simulink model "System_Design_Quadrocopter_2012"  (Simulink 8.1)
settings: Solver=ode45  StartTime=0.0  StopTime=inf  RelTol=1e-3
PostLoadFcn:
  | Reglerauslegung
values from neighbouring files (symbols this model uses):
  f1 = (I_y-I_z)/I_x    [quadrocopter_param.m]
  f2 = rot.J_z/I_x    [quadrocopter_param.m]
  f3 = (I_z-I_x)/I_y    [quadrocopter_param.m]
  f4 = rot.J_z/I_y    [quadrocopter_param.m]
  f5 = (I_x-I_y)/I_z    [quadrocopter_param.m]
  g = 9.81    [quadrocopter_param.m]
  I_x = elec.I_x+bat.I_x+2*boom.I_1x+2*boom.I_1y+2*mot.I_1x+2*mot.I_1y+                             2*rot.I_1x+2*rot.I_1y    [quadrocopter_param.m]
  I_y = elec.I_y+bat.I_y+2*boom.I_1x+2*boom.I_1y+2*mot.I_1x+2*mot.I_1y+                             2*rot.I_1x+2*rot.I_1y    [quadrocopter_param.m]
  I_z = elec.I_z+bat.I_z+4*boom.I_1z+4*mot.I_1z+4*rot.I_1z    [quadrocopter_param.m]
  m = m*1.2    [quadrocopter_param.m]
  r_psi0 = 0    [quadrocopter_param.m]
  r_theta0 = 0    [quadrocopter_param.m]
  theta0 = 0    [quadrocopter_param.m]
  Ts = 0.005    [quadrocopter_param.m]
undefined symbols (not defined in the file or in its folder): boom, K_ret, KV
libraries: Copter_Library x6, simulink x6, dspobslib x4
settings Model: Creator=roczit00  LastModifiedBy=Agrawal
settings DebuggingCC: AlgebraicLoopMsg=none  SolverPrmCheckMsg=none  UnconnectedInputMsg=none  UnconnectedOutputMsg=none  UnconnectedLineMsg=none
settings SFSimCC: SimParseCustomCode=off

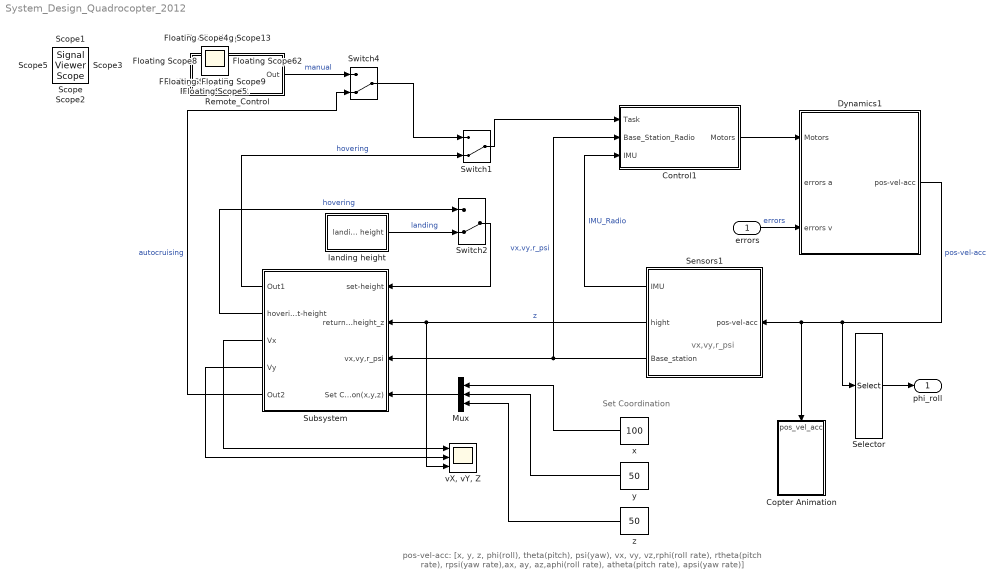
== system System_Design_Quadrocopter_2012 ==
  note: pos-vel-acc: [x, y, z, phi(roll), theta(pitch), psi(yaw), vx, vy, vz,rphi(roll rate), rtheta(pitch rate), rpsi(yaw rate),ax, ay, az,aphi(roll rate), atheta(pitch rate), apsi(yaw rate)]
  note: vx,vy,r_psi
  note: Set Coordination
  errors : Inport
  Control1 : Subsystem
  Copter Animation : Subsystem  mask(Quadrocopter Animation){AXES=[-200 200 -200 200 0 200], T_INT=1/25, K_VAR=Feste Position, K_POS=[200 200 0], K_ANGLE=27, A_ON=on, u_phi=on, u_theta=on, u_psi=on, u_x=on, u_y=on, u_z=on}
      mask prompts: AXES "Achsen Grenzen [xmin xmax ymin ymax zmin zmax]"; T_INT "Zeitintervall zwischen Aktualisierungen [s]:"; K_VAR "Kamera Art:"; K_POS "Ort der Kamera [xc yc zc]:"; K_ANGLE "Öffnungswinkel der Kamera [Grad]:"; A_ON "Animation Einschalten:"; u_phi "Use Input phi:"; u_theta "Use Input theta:"; u_psi "Use Input psi:"; u_x "Use Input x:"; u_y "Use Input y:"; u_z "Use Input z:"
      mask help: Erstellt eine 3-D animierte Ansicht eines Quadrocopters.
      mask init:
      | Config.axes = AXES;
      | Config.update = T_INT;
      | Config.camera_view = K_VAR;
      | Config.camera_pos = K_POS;
      | Config.view = K_ANGLE;
      | Config.Animenable = A_ON;
      | Config.phi = u_phi;
      | Config.theta = u_theta;
      | Config.psi = u_psi;
      | Config.x = u_x;
      | Config.y = u_y;
      | Config.z = u_z;
      mask Help:
      | <p>Dieser Block erstellt ein 3 dimensionales Fenster eines Quadrocopters.
      | 
      | <p><H4>Block Eingänge</H4>
      | Der Eingangsvektor bestehend aus:
      | <ul>
      | <li>X-Koordinate - Ort bezogen auf die X-Achse
      | <li>Y-Koordinate - Ort bezogen auf die Y-Achse
      | <li>Z-Koordinate - Ort bezogen auf die Z-Achse
      | <li>Psi - Yaw Drehung um die Z-Achse
      | <li>Phi - Roll Drehen um die Achse in Flugrichtung
      | <li>theta - pitch Neigung in Flugrichtung nach oben bzw. unten
      | </ul></p>
      mask TypeOptions K_VAR: Feste Position | Frei bewegbar
  Dynamics1 : Subsystem
  Mux : Mux  Inputs=3
  Remote_Control : Subsystem
  Selector : Selector  InputPortWidth=19  IndexOptions=Index vector (dialog)  Indices=[4 5]  OutputSizes=1
  Sensors1 : Subsystem
  Subsystem : Subsystem
  Switch1 : ManualSwitch  CurrentSetting=0
  Switch2 : ManualSwitch  CurrentSetting=0
  Switch4 : ManualSwitch  CurrentSetting=0
  landing height : Subsystem
  "vX, vY, Z" : Scope  NumInputPorts=3
      settings: TimeRange=70  YMin=-5~-10~-20  YMax=25~20~100  SaveName=ScopeData31
  x : Constant  Value=100
  y : Constant  Value=50
  z : Constant  Value=50
  phi_roll : Outport
  Floating Scope{,1..13} (14 alike) : Scope
      Floating Scope settings: Floating=on  YMin=-40  YMax=90
      Floating Scope1 settings: Floating=on
      Floating Scope10 settings: Floating=on  SaveName=ScopeData12
      Floating Scope11 settings: Floating=on  SaveName=ScopeData13
      Floating Scope12 settings: Floating=on  YMin=-2500  YMax=27500  SaveName=ScopeData14
      Floating Scope13 settings: Floating=on  YMin=0  YMax=0.3  SaveName=ScopeData15
      Floating Scope2 settings: Floating=on  YMin=-6000  YMax=2500  SaveName=ScopeData2
      Floating Scope3 settings: Floating=on  SaveName=ScopeData3
      Floating Scope4 settings: Floating=on  SaveName=ScopeData4
      Floating Scope5 settings: Floating=on  YMin=-0.7  YMax=0.8  SaveName=ScopeData5
      Floating Scope6 settings: Floating=on  YMin=-1  YMax=1  SaveName=ScopeData6
      Floating Scope7 settings: Floating=on  YMin=-15  YMax=10  SaveName=ScopeData7
      Floating Scope8 settings: Floating=on  YMax=45  SaveName=ScopeData10
      Floating Scope9 settings: Floating=on  YMin=-7  YMax=9  SaveName=ScopeData11
  Scope{,1..3,5} (5 alike) : SignalViewerScope  IOType=viewer  RefreshTime=0.035000
      Scope settings: YMin=-0.01  YMax=0.1
      Scope2 settings: SaveName=ScopeData2
      Scope3 settings: SaveName=ScopeData3
      Scope5 settings: YMin=0  YMax=275  SaveName=ScopeData4
  wires:
  Dynamics1/1(pos-vel-acc) -> Selector/1, Sensors1/1(pos-vel-acc), Copter Animation/1(pos_vel_acc)  "pos-vel-acc"
  Sensors1/1(IMU) -> Control1/3(IMU)  "IMU_Radio"
  Sensors1/3(Base_station) -> Control1/2(Base_Station_Radio), Subsystem/3(vx,vy,r_psi)  "vx,vy,r_psi"
  errors/1 -> Dynamics1/3(errors v)  "errors"
  Selector/1 -> phi_roll/1
  Control1/1(Motors) -> Dynamics1/1(Motors)
  Subsystem/1(Out1) -> Switch1/2  "hovering"
  Switch1/1 -> Control1/1(Task)
  Sensors1/2(hight) -> Subsystem/2(return height_z), "vX, vY, Z"/3  "z"
  Switch2/1 -> Subsystem/1(set-height)
  Subsystem/3(Vx) -> "vX, vY, Z"/1
  Subsystem/4(Vy) -> "vX, vY, Z"/2
  landing height/1(landing height) -> Switch2/2  "landing"
  Subsystem/2(hovering set-height) -> Switch2/1  "hovering"
  Switch4/1 -> Switch1/1
  Remote_Control/1(Out) -> Switch4/1  "manual"
  Subsystem/5(Out2) -> Switch4/2  "autocruising"
  x/1 -> Mux/1
  y/1 -> Mux/2
  z/1 -> Mux/3
  Mux/1 -> Subsystem/4(Set Coordination(x,y,z))

== system System_Design_Quadrocopter_2012/Control1 ==
  Task : Inport  OutDataTypeStr=double  PortDimensions=4
  Base_Station_Radio : Inport  Port=2
  IMU : Inport  Port=3
  Mux : Mux  Inputs=2
  Mux1 : Mux  Inputs=2
  State Space - 2nd approach : Subsystem
  Motors : Outport  PortDimensions=4
  wires:
  IMU/1 -> Mux/1  "[ax, ay, r_phi, r_theta,r_psi]"
  Task/1 -> Mux/2  "[phi(roll), theta(pitch),rpsi(yaw rate), T(thrust)]"
  Mux/1 -> Mux1/1
  Base_Station_Radio/1 -> Mux1/2  "[vx, vy, rpsi, vz]"
  Mux1/1 -> State Space - 2nd approach/1(In1)
  State Space - 2nd approach/1(Out1) -> Motors/1

== system System_Design_Quadrocopter_2012/Copter Animation ==
  pos_vel_acc : Inport  PortDimensions=19
  S-Function : S-Function  FunctionName=Copter_Animation  Parameters=Config  EnableBusSupport=off
  Selector2 : Selector  InputPortWidth=19  IndexOptions=Index vector (dialog)  Indices=[1 2 3 4 5 6]  OutputSizes=1
  wires:
  pos_vel_acc/1 -> Selector2/1
  Selector2/1 -> S-Function/1

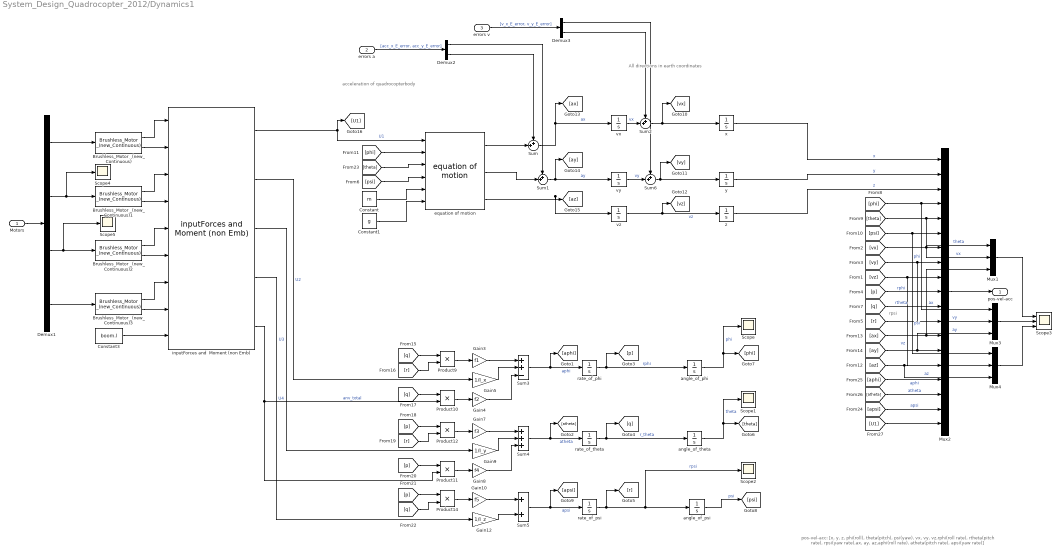
== system System_Design_Quadrocopter_2012/Dynamics1 ==
  note: rpsi
  note: pos-vel-acc: [x, y, z, phi(roll), theta(pitch), psi(yaw), vx, vy, vz,rphi(roll rate), rtheta(pitch rate), rpsi(yaw rate),ax, ay, az,aphi(roll rate), atheta(pitch rate), apsi(yaw rate)]
  note: All directions in earth coordinates
  note: acceleration of quadrocopterbody
  Motors : Inport
  errors a : Inport  Port=2
  errors v : Inport  Port=3
  Brushless_Motor _(new_Continuous){,1..3} (4 alike) : Copter_Library/Brushless_Motor _(new_Continuous)  M_error=0.99
  Constant : Constant  Value=m
  Constant1 : Constant  Value=g
  Constant3 : Constant  Value=boom.l
  Demux1 : Demux
  Demux2 : Demux  Outputs=2
  Demux3 : Demux  Outputs=2
  Gain10 : Gain  Gain=f5
  Gain12 : Gain  Gain=1/I_z
  Gain3 : Gain  Gain=f1
  Gain4 : Gain  Gain=f2
  Gain5 : Gain  Gain=1/I_x
  Gain7 : Gain  Gain=f3
  Gain8 : Gain  Gain=f4
  Gain9 : Gain  Gain=1/I_y
  Mux1 : Mux  Inputs=3
  Mux2 : Mux  Inputs=19
  Mux3 : Mux  Inputs=3
  Mux4 : Mux  Inputs=3
  Product{9..12,14} (5 alike) : Product  RndMeth=Zero
  Scope{,1..2,4..5} (5 alike) : Scope
      Scope settings: YMin=-1  YMax=1  SaveName=ScopeData8
      Scope1 settings: YMin=-54  YMax=-49.5  SaveName=ScopeData9
      Scope2 settings: YMin=17.1  YMax=19.1  SaveName=ScopeData16
      Scope4 settings: YMin=-1  YMax=260  SaveName=ScopeData18
      Scope5 settings: YMin=-1  YMax=260  SaveName=ScopeData19
  Scope3 : Scope  NumInputPorts=3
      settings: TimeRange=10  YMin=-5~-5~-10  YMax=8~7~40  SaveName=ScopeData29
  Sum{,1..2,6} (4 alike) : Sum  Inputs=++|
  Sum3 : Sum  Inputs=++-
  Sum4 : Sum  Inputs=+++
  Sum5 : Sum
  angle_of_phi : Integrator
  angle_of_psi : Integrator
  angle_of_theta : Integrator  InitialCondition=theta0
  equation of motion : Copter_Library/equation of motion
  inputForces and  Moment (non Emb) : Copter_Library/inputForces and  Moment (non Emb)
  rate_of_phi : Integrator
  rate_of_psi : Integrator  InitialCondition=r_psi0
  rate_of_theta : Integrator  InitialCondition=r_theta0
  vx : Integrator
  vy : Integrator
  vz : Integrator
  x : Integrator
  y : Integrator
  z : Integrator
  pos-vel-acc : Outport
  wires:
  [apsi] -> Mux2/18  "apsi"
  [atheta] -> Mux2/17  "atheta"
  [aphi] -> Mux2/16  "aphi"
  [az] -> Mux2/15, Mux4/3  "az"
  [ay] -> Mux2/14, Mux3/3  "ay"
  [ax] -> Mux2/13, Mux1/3  "ax"
  [r] -> Mux2/12
  [q] -> Mux2/11  "rtheta"
  [p] -> Mux2/10  "rphi"
  [vz] -> Mux2/9, Mux4/2  "vz"
  [vy] -> Mux2/8, Mux3/2  "vy"
  [vx] -> Mux2/7, Mux1/2  "vx"
  [psi] -> Mux2/6, Mux4/1  "psi"
  [theta] -> Mux2/5, Mux1/1  "theta"
  [phi] -> Mux2/4, Mux3/1  "phi"
  z/1 -> Mux2/3  "z"
  Mux2/1 -> pos-vel-acc/1
  errors a/1 -> Demux2/1  "[acc_x_E_error, acc_y_E_error]"
  Motors/1 -> Demux1/1
  Demux1/3 -> Brushless_Motor _(new_Continuous)2/1, Scope5/1
  Demux1/4 -> Brushless_Motor _(new_Continuous)3/1
  Demux1/2 -> Brushless_Motor _(new_Continuous)1/1, Scope4/1
  Demux1/1 -> Brushless_Motor _(new_Continuous)/1
  vz/1 -> [vz], z/1  "vz"
  Constant3/1 -> inputForces and  Moment (non Emb)/9
  Sum5/1 -> [apsi], rate_of_psi/1  "apsi"
  inputForces and  Moment (non Emb)/4 -> Gain12/1  "U4"
  Gain12/1 -> Sum5/2
  Gain10/1 -> Sum5/1
  Product14/1 -> Gain10/1
  [q] -> Product14/2
  [p] -> Product14/1
  Sum4/1 -> [atheta], rate_of_theta/1  "atheta"
  inputForces and  Moment (non Emb)/3 -> Gain9/1  "U3"
  Gain8/1 -> Sum4/3
  Gain9/1 -> Sum4/2
  Product11/1 -> Gain8/1
  [p] -> Product11/1
  Gain7/1 -> Sum4/1
  Product12/1 -> Gain7/1
  [r] -> Product12/2
  [p] -> Product12/1
  Sum3/1 -> [aphi], rate_of_phi/1  "aphi"
  Gain4/1 -> Sum3/3
  Gain5/1 -> Sum3/2
  inputForces and  Moment (non Emb)/2 -> Gain5/1  "U2"
  Product10/1 -> Gain4/1
  [q] -> Product10/1
  Gain3/1 -> Sum3/1
  Product9/1 -> Gain3/1
  [r] -> Product9/2
  [q] -> Product9/1
  inputForces and  Moment (non Emb)/5 -> Product11/2, Product10/2  "anv_total"
  angle_of_phi/1 -> [phi], Scope/1  "phi"
  angle_of_theta/1 -> [theta], Scope1/1  "theta"
  angle_of_psi/1 -> [psi]  "psi"
  rate_of_phi/1 -> [p], angle_of_phi/1  "rphi"
  rate_of_theta/1 -> angle_of_theta/1, [q]  "r_theta"
  rate_of_psi/1 -> [r], angle_of_psi/1, Scope2/1  "rpsi"
  Brushless_Motor _(new_Continuous)/1 -> inputForces and  Moment (non Emb)/1
  Brushless_Motor _(new_Continuous)/2 -> inputForces and  Moment (non Emb)/2
  Brushless_Motor _(new_Continuous)1/1 -> inputForces and  Moment (non Emb)/3
  Brushless_Motor _(new_Continuous)1/2 -> inputForces and  Moment (non Emb)/4
  Brushless_Motor _(new_Continuous)2/1 -> inputForces and  Moment (non Emb)/5
  Brushless_Motor _(new_Continuous)2/2 -> inputForces and  Moment (non Emb)/6
  Brushless_Motor _(new_Continuous)3/1 -> inputForces and  Moment (non Emb)/7
  Brushless_Motor _(new_Continuous)3/2 -> inputForces and  Moment (non Emb)/8
  x/1 -> Mux2/1  "x"
  y/1 -> Mux2/2  "y"
  Sum1/1 -> [ay], vy/1  "ay"
  Sum/1 -> [ax], vx/1  "ax"
  Demux2/2 -> Sum/1
  Demux2/1 -> Sum1/1
  equation of motion/3 -> [az], vz/1
  equation of motion/2 -> Sum1/2
  equation of motion/1 -> Sum/2
  inputForces and  Moment (non Emb)/1 -> [U1], equation of motion/1  "U1"
  [phi] -> equation of motion/2
  [theta] -> equation of motion/3
  [psi] -> equation of motion/4
  Constant/1 -> equation of motion/5
  Constant1/1 -> equation of motion/6
  [U1] -> Mux2/19
  errors v/1 -> Demux3/1  "[v_x_E_error, v_y_E_error]"
  Demux3/2 -> Sum2/1
  Demux3/1 -> Sum6/1
  vx/1 -> Sum2/2  "vx"
  Sum2/1 -> [vx], x/1
  vy/1 -> Sum6/2  "vy"
  Sum6/1 -> [vy], y/1
  Mux1/1 -> Scope3/1
  Mux3/1 -> Scope3/2
  Mux4/1 -> Scope3/3

== system System_Design_Quadrocopter_2012/Remote_Control ==
  3D-Mouse : ManualSwitch  CurrentSetting=0
  Allow 3D Mouse : dspobslib/DSP Constant  Value=1  SampleMode=Discrete  discreteOutput=Sample-based  continuousOutput=Sample-based  sampTime=inf  framePeriod=2  dataType=boolean  isSigned=on  wordLen=16  udDataType=sfix(16)  fracBitsMode=Best precision  numFracBits=15  InterpretAs1D=-inf  Ts=-inf  FramebasedOutput=-inf
  Disable 3D Mouse : dspobslib/DSP Constant  Value=0  SampleMode=Discrete  discreteOutput=Sample-based  continuousOutput=Sample-based  sampTime=inf  framePeriod=2  dataType=boolean  isSigned=on  wordLen=16  udDataType=sfix(16)  fracBitsMode=Best precision  numFracBits=15  InterpretAs1D=-inf  Ts=-inf  FramebasedOutput=-inf
  Manual Switch2 : ManualSwitch
  Remote_Control_3d_mouse : Subsystem  AncestorBlock=Remote_Control_Library/Remote_Control_3d_mouse
  Remote_Control_setting : Subsystem  AncestorBlock=Remote_Control_Library/Remote_Control_Pitch_stimuli
  Out : Outport
  wires:
  Remote_Control_setting/1(Out) -> Manual Switch2/1
  Manual Switch2/1 -> Out/1
  Allow 3D Mouse/1 -> 3D-Mouse/1
  Disable 3D Mouse/1 -> 3D-Mouse/2
  3D-Mouse/1 -> Remote_Control_3d_mouse/Enable
  Remote_Control_3d_mouse/1(Out1) -> Manual Switch2/2

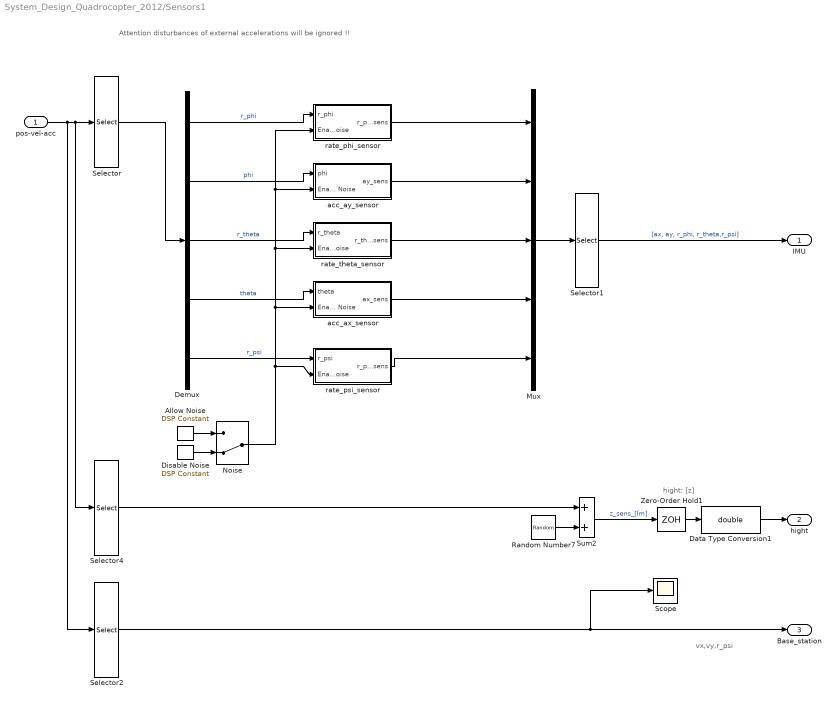
== system System_Design_Quadrocopter_2012/Sensors1 ==
  note: Attention disturbances of external accelerations will be ignored !!
  note: hight: [z]
  note: vx,vy,r_psi
  pos-vel-acc : Inport  PortDimensions=19
  Allow Noise : dspobslib/DSP Constant  Value=1  SampleMode=Discrete  discreteOutput=Sample-based  continuousOutput=Sample-based  sampTime=inf  framePeriod=2  dataType=boolean  isSigned=on  wordLen=16  udDataType=sfix(16)  fracBitsMode=Best precision  numFracBits=15  InterpretAs1D=-inf  Ts=-inf  FramebasedOutput=-inf
  Data Type Conversion1 : DataTypeConversion  OutDataTypeStr=double  RndMeth=Round
  Demux : Demux  Outputs=5
  Disable Noise : dspobslib/DSP Constant  Value=0  SampleMode=Discrete  discreteOutput=Sample-based  continuousOutput=Sample-based  sampTime=inf  framePeriod=2  dataType=boolean  isSigned=on  wordLen=16  udDataType=sfix(16)  fracBitsMode=Best precision  numFracBits=15  InterpretAs1D=-inf  Ts=-inf  FramebasedOutput=-inf
  Mux : Mux  Inputs=5
  Noise : ManualSwitch  CurrentSetting=0
  Random Number7 : RandomNumber  Variance=3.0462e-8  Seed=5756  SampleTime=0.01
  Scope : Scope
      settings: SaveName=ScopeData30
  Selector : Selector  InputPortWidth=19  IndexOptions=Index vector (dialog)  Indices=[10 4 11 5 12]  OutputSizes=1
  Selector1 : Selector  InputPortWidth=5  IndexOptions=Index vector (dialog)  Indices=[4 2 1 3 5]  OutputSizes=1
  Selector2 : Selector  InputPortWidth=19  IndexOptions=Index vector (dialog)  Indices=[7 8 12]  OutputSizes=1
  Selector4 : Selector  InputPortWidth=19  IndexOptions=Index vector (dialog)  Indices=[3]  OutputSizes=1
  Sum2 : Sum
  Zero-Order Hold1 : ZeroOrderHold  SampleTime=Ts
  acc_ax_sensor : Subsystem
  acc_ay_sensor : Subsystem
  rate_phi_sensor : Subsystem
  rate_psi_sensor : Subsystem
  rate_theta_sensor : Subsystem
  IMU : Outport
  hight : Outport  Port=2
  Base_station : Outport  Port=3
  wires:
  pos-vel-acc/1 -> Selector/1, Selector4/1, Selector2/1
  Selector/1 -> Demux/1
  rate_phi_sensor/1(r_phi_sens) -> Mux/1
  acc_ay_sensor/1(ay_sens) -> Mux/2
  rate_theta_sensor/1(r_theta_sens) -> Mux/3
  acc_ax_sensor/1(ax_sens) -> Mux/4
  rate_psi_sensor/1(r_psi_sens) -> Mux/5
  Demux/1 -> rate_phi_sensor/1(r_phi)  "r_phi"
  Demux/2 -> acc_ay_sensor/1(phi)  "phi"
  Demux/3 -> rate_theta_sensor/1(r_theta)  "r_theta"
  Demux/4 -> acc_ax_sensor/1(theta)  "theta"
  Demux/5 -> rate_psi_sensor/1(r_psi)  "r_psi"
  Mux/1 -> Selector1/1
  Selector1/1 -> IMU/1  "[ax, ay, r_phi, r_theta,r_psi]"
  Allow Noise/1 -> Noise/1
  Disable Noise/1 -> Noise/2
  Noise/1 -> rate_psi_sensor/2(Enable Noise), acc_ax_sensor/2(Enable Noise), rate_theta_sensor/2(Enable Noise), acc_ay_sensor/2(Enable Noise), rate_phi_sensor/2(Enable Noise)
  Random Number7/1 -> Sum2/2
  Selector4/1 -> Sum2/1
  Sum2/1 -> Zero-Order Hold1/1  "z_sens_[Ïm]"
  Zero-Order Hold1/1 -> Data Type Conversion1/1
  Data Type Conversion1/1 -> hight/1
  Selector2/1 -> Base_station/1, Scope/1

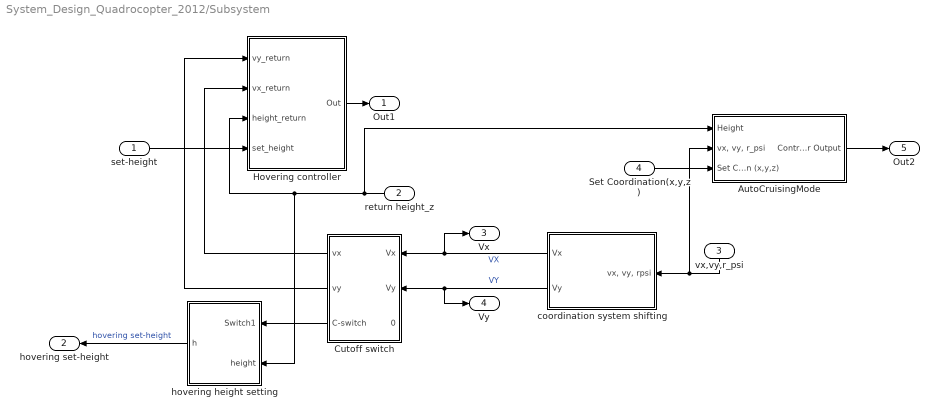
== system System_Design_Quadrocopter_2012/Subsystem ==
  set-height : Inport
  return height_z : Inport  Port=2
  vx,vy,r_psi : Inport  Port=3
  Set Coordination(x,y,z) : Inport  Port=4
  AutoCruisingMode : Subsystem
  Cutoff switch : Subsystem
  Hovering controller : Subsystem
  coordination system shifting : Subsystem
  hovering height setting : MATLAB Function  TreatAsAtomicUnit=on
  Out1 : Outport
  hovering set-height : Outport  Port=2
  Vx : Outport  Port=3
  Vy : Outport  Port=4
  Out2 : Outport  Port=5
  wires:
  Cutoff switch/3(C-switch) -> hovering height setting/1(Switch1)
  coordination system shifting/2(Vy) -> Cutoff switch/2(Vy), Vy/1  "VY"
  Cutoff switch/1(vx) -> Hovering controller/2(vx_return)
  Cutoff switch/2(vy) -> Hovering controller/1(vy_return)
  return height_z/1 -> Hovering controller/3(height_return), hovering height setting/2(height), AutoCruisingMode/1(Height)
  vx,vy,r_psi/1 -> coordination system shifting/1("vx, vy, rpsi"), AutoCruisingMode/2("vx, vy, r_psi")
  Hovering controller/1(Out) -> Out1/1
  set-height/1 -> Hovering controller/4(set_height)
  hovering height setting/1(h) -> hovering set-height/1  "hovering set-height"
  coordination system shifting/1(Vx) -> Cutoff switch/1(Vx), Vx/1  "VX"
  AutoCruisingMode/1(Controller Output) -> Out2/1
  Set Coordination(x,y,z)/1 -> AutoCruisingMode/3(Set Coordination (x,y,z))

== system System_Design_Quadrocopter_2012/landing height ==
  Add1 : Sum
  Compensate height : Constant  Value=5
  landing set_height : Constant  Value=10
  landing height : Outport
  wires:
  landing set_height/1 -> Add1/2
  Compensate height/1 -> Add1/1
  Add1/1 -> landing height/1

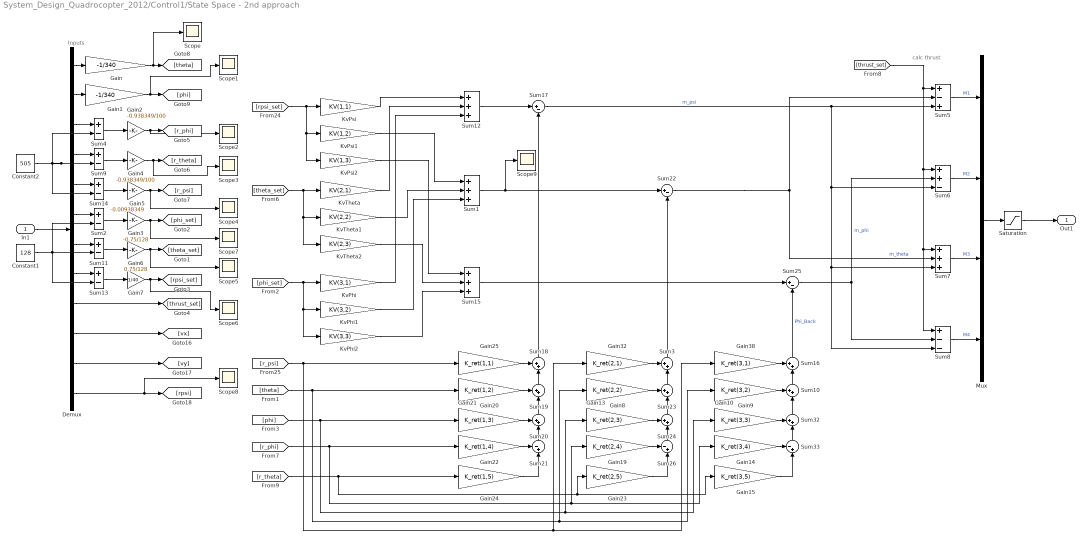
== system System_Design_Quadrocopter_2012/Control1/State Space - 2nd approach ==
  note: calc thrust
  note: Inputs
  In1 : Inport
  Constant1 : Constant  Value=128
  Constant2 : Constant  Value=505
  Demux : Demux  Outputs=12
  Gain : Gain  Gain=-1/340
  Gain1 : Gain  Gain=-1/340
  Gain10 : Gain  Gain=K_ret(3,3)
  Gain13 : Gain  Gain=K_ret(2,3)
  Gain14 : Gain  Gain=K_ret(3,4)
  Gain15 : Gain  Gain=K_ret(3,5)
  Gain19 : Gain  Gain=K_ret(2,4)
  Gain2 : Gain  Gain=-0.938349/100
  Gain20 : Gain  Gain=K_ret(1,2)
  Gain21 : Gain  Gain=K_ret(1,3)
  Gain22 : Gain  Gain=K_ret(1,4)
  Gain23 : Gain  Gain=K_ret(2,5)
  Gain24 : Gain  Gain=K_ret(1,5)
  Gain25 : Gain  Gain=K_ret(1,1)
  Gain3 : Gain  Gain=-0.75/128
  Gain32 : Gain  Gain=K_ret(2,1)
  Gain38 : Gain  Gain=K_ret(3,1)
  Gain4 : Gain  Gain=-0.938349/100
  Gain5 : Gain  Gain=-0.00938349
  Gain6 : Gain  Gain=0.75/128
  Gain7 : Gain  Gain=1/40
  Gain8 : Gain  Gain=K_ret(2,2)
  Gain9 : Gain  Gain=K_ret(3,2)
  KvPhi : Gain  Gain=KV(3,1)
  KvPhi1 : Gain  Gain=KV(3,2)
  KvPhi2 : Gain  Gain=KV(3,3)
  KvPsi : Gain  Gain=KV(1,1)
  KvPsi1 : Gain  Gain=KV(1,2)
  KvPsi2 : Gain  Gain=KV(1,3)
  KvTheta : Gain  Gain=KV(2,1)
  KvTheta1 : Gain  Gain=KV(2,2)
  KvTheta2 : Gain  Gain=KV(2,3)
  Mux : Mux
  Saturation : Saturate  UpperLimit=255  LowerLimit=0
  Scope{,1..9} (10 alike) : Scope
      Scope settings: SaveName=ScopeData17
      Scope1 settings: SaveName=ScopeData20
      Scope2 settings: SaveName=ScopeData21
      Scope3 settings: SaveName=ScopeData22
      Scope4 settings: SaveName=ScopeData23
      Scope5 settings: SaveName=ScopeData24
      Scope6 settings: SaveName=ScopeData25
      Scope7 settings: SaveName=ScopeData26
      Scope8 settings: SaveName=ScopeData27
      Scope9 settings: SaveName=ScopeData28
  Sum{1,7,12,15} (4 alike) : Sum  Inputs=+++
  Sum{3,10,16,18..20,23..24,32} (9 alike) : Sum  Inputs=++|
  Sum{2,4,9,11,13..14} (6 alike) : Sum  Inputs=+-
  Sum17 : Sum  Inputs=|+-
  Sum21 : Sum  Inputs=-+|
  Sum22 : Sum  Inputs=|+-
  Sum25 : Sum  Inputs=|+-
  Sum26 : Sum  Inputs=-+|
  Sum33 : Sum  Inputs=-+|
  Sum5 : Sum  Inputs=+-+
  Sum6 : Sum  Inputs=++-
  Sum8 : Sum  Inputs=+--
  Out1 : Outport
  wires:
  Saturation/1 -> Out1/1
  Mux/1 -> Saturation/1
  [thrust_set] -> Sum8/1, Sum7/1, Sum6/1, Sum5/1
  Sum25/1 -> Sum6/2, Sum8/2  "m_phi"
  Sum6/1 -> Mux/2  "M2"
  Sum7/1 -> Mux/3  "M3"
  Sum8/1 -> Mux/4  "M4"
  Sum5/1 -> Mux/1  "M1"
  Gain1/1 -> [phi], Scope1/1
  Gain/1 -> [theta], Scope/1
  Demux/9 -> [thrust_set]
  Demux/1 -> Gain/1
  Demux/2 -> Gain1/1
  In1/1 -> Demux/1
  Demux/10 -> [vx]
  Demux/11 -> [vy]
  Demux/12 -> [rpsi], Scope8/1
  Sum17/1 -> Sum5/3, Sum6/3, Sum7/3, Sum8/3  "m_psi"
  [phi_set] -> KvPhi/1, KvPhi1/1, KvPhi2/1
  [rpsi_set] -> KvPsi/1, KvPsi2/1, KvPsi1/1
  Demux/3 -> Sum4/1
  Sum4/1 -> Gain2/1
  Constant2/1 -> Sum4/2, Sum9/2, Sum14/2
  Gain2/1 -> [r_phi], Scope2/1
  Demux/4 -> Sum9/1
  Sum9/1 -> Gain4/1
  Gain4/1 -> [r_theta], Scope3/1
  Gain5/1 -> [r_psi], Scope4/1
  Demux/5 -> Sum14/1
  Sum14/1 -> Gain5/1
  KvPsi/1 -> Sum12/1
  KvTheta/1 -> Sum12/2
  KvPhi/1 -> Sum12/3
  KvPsi1/1 -> Sum1/1
  KvTheta1/1 -> Sum1/2
  KvPhi1/1 -> Sum1/3
  KvPhi2/1 -> Sum15/3
  KvTheta2/1 -> Sum15/2
  KvPsi2/1 -> Sum15/1
  [theta_set] -> KvTheta/1, KvTheta1/1, KvTheta2/1
  Gain3/1 -> [phi_set], Scope7/1
  Demux/6 -> Sum2/1
  Sum2/1 -> Gain3/1
  Constant1/1 -> Sum2/2, Sum13/2, Sum11/2
  Gain7/1 -> [rpsi_set], Scope6/1
  Gain6/1 -> [theta_set], Scope5/1
  Sum11/1 -> Gain6/1
  Sum13/1 -> Gain7/1
  Demux/8 -> Sum13/1
  Demux/7 -> Sum11/1
  Gain8/1 -> Sum23/1
  Sum24/1 -> Sum23/2
  Sum23/1 -> Sum3/2
  Sum26/1 -> Sum24/2
  Gain23/1 -> Sum26/2
  Sum32/1 -> Sum10/2
  Sum10/1 -> Sum16/2
  Sum33/1 -> Sum32/2
  Gain19/1 -> Sum26/1
  Gain13/1 -> Sum24/1
  Gain32/1 -> Sum3/1
  Gain38/1 -> Sum16/1
  Gain9/1 -> Sum10/1
  Gain10/1 -> Sum32/1
  Gain14/1 -> Sum33/1
  Gain15/1 -> Sum33/2
  Gain25/1 -> Sum18/1
  Sum20/1 -> Sum19/2
  Sum19/1 -> Sum18/2
  Sum21/1 -> Sum20/2
  Gain24/1 -> Sum21/2
  Gain22/1 -> Sum21/1
  Gain21/1 -> Sum20/1
  Gain20/1 -> Sum19/1
  [r_psi] -> Gain25/1, Gain32/1, Gain38/1
  [theta] -> Gain20/1, Gain8/1, Gain9/1
  [phi] -> Gain21/1, Gain13/1, Gain10/1
  [r_phi] -> Gain22/1, Gain19/1, Gain14/1
  [r_theta] -> Gain24/1, Gain23/1, Gain15/1
  Sum12/1 -> Sum17/1
  Sum18/1 -> Sum17/2
  Sum1/1 -> Sum22/1, Scope9/1
  Sum3/1 -> Sum22/2
  Sum22/1 -> Sum7/2, Sum5/2  "m_theta"
  Sum16/1 -> Sum25/2  "Phi_Back"
  Sum15/1 -> Sum25/1

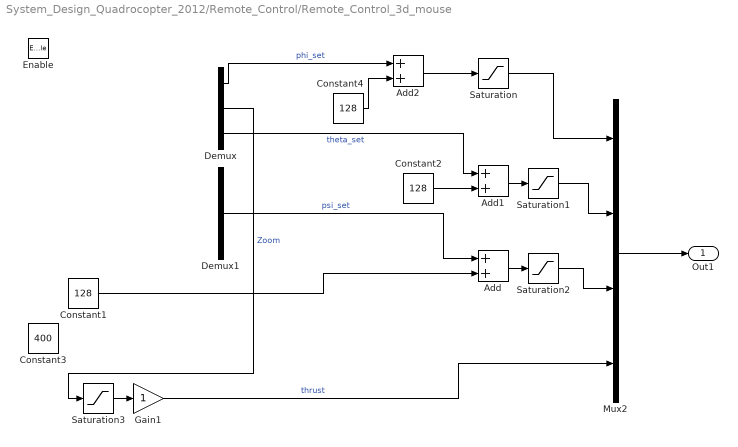
== system System_Design_Quadrocopter_2012/Remote_Control/Remote_Control_3d_mouse ==
  Enable : EnablePort  PropagateVarSize=During execution
  Add : Sum
  Add1 : Sum
  Add2 : Sum
  Constant1 : Constant  Value=128
  Constant2 : Constant  Value=128
  Constant3 : Constant  Value=400
  Constant4 : Constant  Value=128
  Demux : Demux  Outputs=3
  Demux1 : Demux  Outputs=3
  Gain1 : Gain
  Mux2 : Mux
  Saturation : Saturate  UpperLimit=255  LowerLimit=0
  Saturation1 : Saturate  UpperLimit=255  LowerLimit=0
  Saturation2 : Saturate  UpperLimit=255  LowerLimit=0
  Saturation3 : Saturate  UpperLimit=inf  LowerLimit=0
  Out1 : Outport
  wires:
  Demux/1 -> Add2/1  "phi_set"
  Constant4/1 -> Add2/2
  Demux/3 -> Add1/1  "theta_set"
  Constant2/1 -> Add1/2
  Add/1 -> Saturation2/1
  Demux1/2 -> Add/1  "psi_set"
  Constant1/1 -> Add/2
  ? -> Demux1/1  "[Kippen, Rollen, Drehen]"
  ? -> Demux/1  "[Trans_X, Trans_Z, Trans_Y]"
  Gain1/1 -> Mux2/4  "thrust"
  Mux2/1 -> Out1/1
  Add2/1 -> Saturation/1
  Add1/1 -> Saturation1/1
  Saturation1/1 -> Mux2/2
  Saturation2/1 -> Mux2/3
  Saturation/1 -> Mux2/1
  Saturation3/1 -> Gain1/1
  Demux/2 -> Saturation3/1  "Zoom"

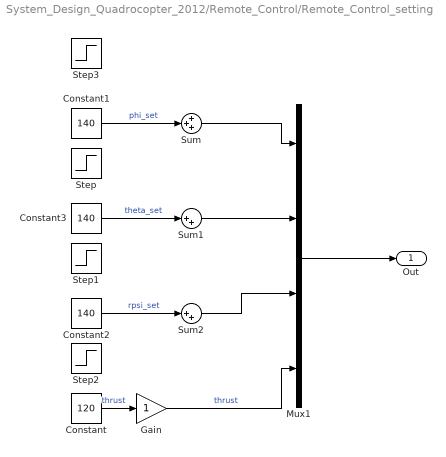
== system System_Design_Quadrocopter_2012/Remote_Control/Remote_Control_setting ==
  Constant : Constant  Value=120
  Constant1 : Constant  Value=140
  Constant2 : Constant  Value=140
  Constant3 : Constant  Value=140
  Gain : Gain
  Mux1 : Mux
  Step : Step  After=0  SampleTime=0
  Step1 : Step  After=50  SampleTime=0
  Step2 : Step  After=50  SampleTime=0
  Step3 : Step  After=50  SampleTime=0
  Sum : Sum  Inputs=+++
  Sum1 : Sum  Inputs=|++
  Sum2 : Sum  Inputs=|++
  Out : Outport
  wires:
  Constant/1 -> Gain/1  "thrust"
  Mux1/1 -> Out/1
  Gain/1 -> Mux1/4  "thrust"
  Sum/1 -> Mux1/1
  Constant3/1 -> Sum1/1  "theta_set"
  Sum1/1 -> Mux1/2
  Constant2/1 -> Sum2/1  "rpsi_set"
  Sum2/1 -> Mux1/3
  Constant1/1 -> Sum/2  "phi_set"

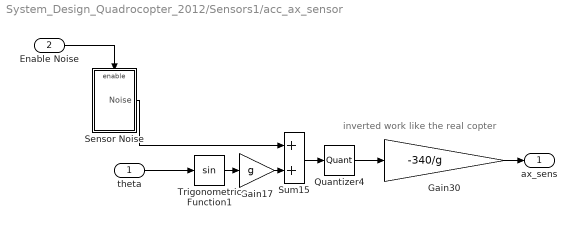
== system System_Design_Quadrocopter_2012/Sensors1/acc_ax_sensor ==
  note: inverted work like the real copter
  theta : Inport
  Enable Noise : Inport  Port=2
  Gain17 : Gain  Gain=g
  Gain30 : Gain  Gain=-340/g
  Quantizer4 : Quantizer  QuantizationInterval=g/340  SampleTime=Ts
  Sensor Noise : Subsystem
  Sum15 : Sum
  Trigonometric Function1 : Trigonometry
  ax_sens : Outport
  wires:
  Sensor Noise/1(Noise) -> Sum15/1
  Sum15/1 -> Quantizer4/1
  Trigonometric Function1/1 -> Gain17/1
  Gain17/1 -> Sum15/2
  Quantizer4/1 -> Gain30/1
  theta/1 -> Trigonometric Function1/1
  Gain30/1 -> ax_sens/1
  Enable Noise/1 -> Sensor Noise/Enable

== system System_Design_Quadrocopter_2012/Sensors1/acc_ay_sensor ==
  note: inverted like in the real copter
  phi : Inport
  Enable Noise : Inport  Port=2
  Gain19 : Gain  Gain=-340/g
  Gain22 : Gain  Gain=g
  Quantizer3 : Quantizer  QuantizationInterval=g/340  SampleTime=Ts
  Sensor Noise : Subsystem
  Sum12 : Sum
  Trigonometric Function : Trigonometry
  ay_sens : Outport
  wires:
  Sum12/1 -> Quantizer3/1
  Trigonometric Function/1 -> Gain22/1
  Gain22/1 -> Sum12/2
  Quantizer3/1 -> Gain19/1
  phi/1 -> Trigonometric Function/1
  Gain19/1 -> ay_sens/1
  Enable Noise/1 -> Sensor Noise/Enable
  Sensor Noise/1(Noise) -> Sum12/1

== system System_Design_Quadrocopter_2012/Sensors1/rate_phi_sensor ==
  note: Sensor adds noise and Samples and quantize the Signal. In combination with the gain a integer value is generated
      | like the Sensor is read from the ADC registers.
  r_phi : Inport
  Enable Noise : Inport  Port=2
  Gain20 : Gain  Gain=1/0.00938349
  Offset : Constant  Value=505
  Quantizer : Quantizer  QuantizationInterval=0.00938349  SampleTime=Ts
  Sensor Noise : Subsystem
  Sum : Sum  Inputs=++|
  Sum14 : Sum
  r_phi_sens : Outport
  wires:
  Sum14/1 -> Quantizer/1
  Quantizer/1 -> Gain20/1
  r_phi/1 -> Sum14/2
  Gain20/1 -> Sum/2
  Offset/1 -> Sum/1
  Sum/1 -> r_phi_sens/1
  Enable Noise/1 -> Sensor Noise/Enable
  Sensor Noise/1(Noise) -> Sum14/1

== system System_Design_Quadrocopter_2012/Sensors1/rate_psi_sensor ==
  note: inverted to simulate real copter
  r_psi : Inport
  Enable Noise : Inport  Port=2
  Gain25 : Gain  Gain=-1/0.00938349
  Offset : Constant  Value=505
  Quantizer2 : Quantizer  QuantizationInterval=0.00938349  SampleTime=Ts
  Sensor Noise : Subsystem
  Sum : Sum  Inputs=++|
  Sum13 : Sum
  r_psi_sens : Outport
  wires:
  Sensor Noise/1(Noise) -> Sum13/1
  Sum13/1 -> Quantizer2/1
  Quantizer2/1 -> Gain25/1
  r_psi/1 -> Sum13/2
  Offset/1 -> Sum/1
  Gain25/1 -> Sum/2
  Sum/1 -> r_psi_sens/1
  Enable Noise/1 -> Sensor Noise/Enable

== system System_Design_Quadrocopter_2012/Sensors1/rate_theta_sensor ==
  note: inverted to worj like in the real copter
  r_theta : Inport
  Enable Noise : Inport  Port=2
  Gain27 : Gain  Gain=-1/0.00938349
  Offset : Constant  Value=505
  Quantizer1 : Quantizer  QuantizationInterval=0.00938349  SampleTime=Ts
  Sensor Noise : Subsystem
  Sum : Sum  Inputs=++|
  Sum16 : Sum
  r_theta_sens : Outport
  wires:
  Sum16/1 -> Quantizer1/1
  Quantizer1/1 -> Gain27/1
  r_theta/1 -> Sum16/2
  Offset/1 -> Sum/1
  Gain27/1 -> Sum/2
  Sum/1 -> r_theta_sens/1
  Enable Noise/1 -> Sensor Noise/Enable
  Sensor Noise/1(Noise) -> Sum16/1

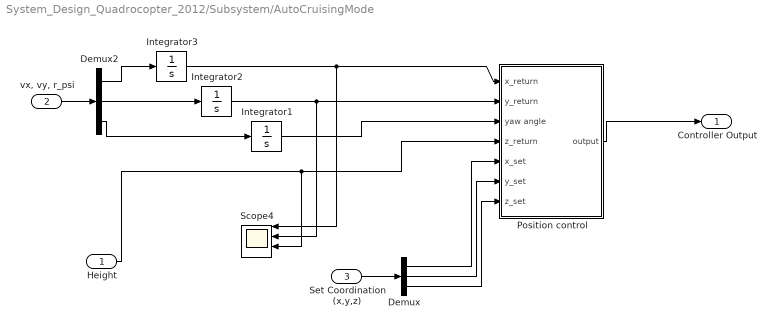
== system System_Design_Quadrocopter_2012/Subsystem/AutoCruisingMode ==
  Height : Inport
  "vx, vy, r_psi" : Inport  Port=2
  Set Coordination (x,y,z) : Inport  Port=3
  Demux : Demux  Outputs=3
  Demux2 : Demux  Outputs=3
  Integrator1 : Integrator
  Integrator2 : Integrator
  Integrator3 : Integrator
  Position control : Subsystem
  Scope4 : Scope  NumInputPorts=4
      settings: TimeRange=100  YMin=1.775~2.125~-26000~-1  YMax=1.975~2.375~-21500~1  SaveName=ScopeData31
  Controller Output : Outport
  wires:
  "vx, vy, r_psi"/1 -> Demux2/1
  Position control/1(output) -> Controller Output/1
  Height/1 -> Position control/4(z_return), Scope4/3
  Demux2/1 -> Integrator3/1
  Demux2/2 -> Integrator2/1
  Demux2/3 -> Integrator1/1
  Integrator3/1 -> Position control/1(x_return), Scope4/1
  Integrator2/1 -> Scope4/2, Position control/2(y_return)
  Integrator1/1 -> Position control/3(yaw angle)
  Set Coordination (x,y,z)/1 -> Demux/1
  Demux/1 -> Position control/5(x_set)
  Demux/2 -> Position control/6(y_set)
  Demux/3 -> Position control/7(z_set)

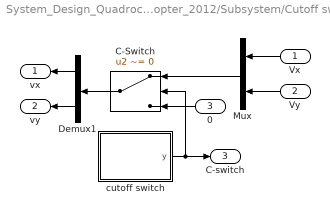
== system System_Design_Quadrocopter_2012/Subsystem/Cutoff switch ==
  Vx : Inport
  Vy : Inport  Port=2
  0 : Inport  Port=3
  C-Switch : Switch  Criteria=u2 ~= 0
  Demux1 : Demux  Outputs=2
  Mux : Mux  Inputs=2
  cutoff switch : MATLAB Function  TreatAsAtomicUnit=on
  vx : Outport
  vy : Outport  Port=2
  C-switch : Outport  Port=3
  wires:
  cutoff switch/1(y) -> C-Switch/2, C-switch/1
  C-Switch/1 -> Demux1/1
  Mux/1 -> C-Switch/1
  Vx/1 -> Mux/1
  Vy/1 -> Mux/2
  Demux1/1 -> vx/1
  Demux1/2 -> vy/1
  0/1 -> C-Switch/3

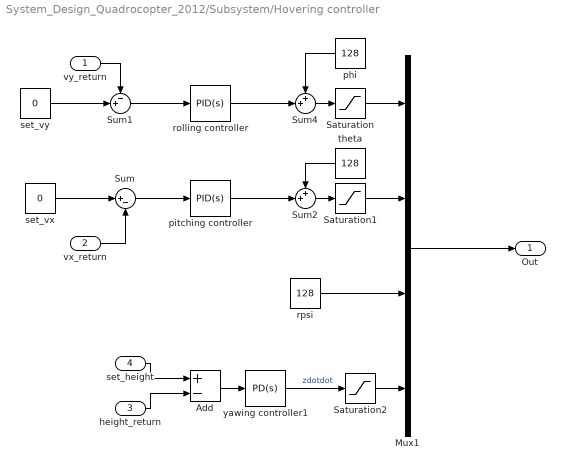
== system System_Design_Quadrocopter_2012/Subsystem/Hovering controller ==
  vy_return : Inport
  vx_return : Inport  Port=2
  height_return : Inport  Port=3
  set_height : Inport  Port=4
  " rolling controller" : simulink/Continuous/PID Controller  Controller=PID  TimeDomain=Continuous-time  SampleTime=1  IntegratorMethod=Forward Euler  FilterMethod=Forward Euler  Form=Parallel  P=25  I=10  D=20  N=100  InitialConditionSource=internal  InitialConditionForIntegrator=0  InitialConditionForFilter=0  ExternalReset=none  LimitOutput=on  UpperSaturationLimit=128  LowerSaturationLimit=-128  LinearizeAsGain=off  AntiWindupMode=clamping  Kb=1  TrackingMode=off  Kt=1  PParamMin=[]  PParamMax=[]  IParamMin=[]  IParamMax=[]  DParamMin=[]  DParamMax=[]  NParamMin=[]  NParamMax=[]  KbParamMin=[]  KbParamMax=[]  KtParamMin=[]  KtParamMax=[]  POutMin=[]  POutMax=[]  IOutMin=[]  IOutMax=[]  DOutMin=[]  DOutMax=[]  NOutMin=[]  NOutMax=[]  KbOutMin=[]  KbOutMax=[]  KtOutMin=[]  KtOutMax=[]  IntegratorOutMin=[]  IntegratorOutMax=[]  FilterOutMin=[]  FilterOutMax=[]  SumOutMin=[]  SumOutMax=[]  SumI1OutMin=[]  SumI1OutMax=[]  SumI2OutMin=[]  SumI2OutMax=[]  SumI3OutMin=[]  SumI3OutMax=[]  SumDOutMin=[]  SumDOutMax=[]  SaturationOutMin=[]  SaturationOutMax=[]  IntegratorContinuousStateAttributes=''  IntegratorStateMustResolveToSignalObject=off  IntegratorRTWStateStorageClass=Auto  FilterContinuousStateAttributes=''  FilterStateMustResolveToSignalObject=off  FilterRTWStateStorageClass=Auto
  Add : Sum  Inputs=+-
  Mux1 : Mux
  Saturation : Saturate  UpperLimit=255  LowerLimit=0
  Saturation1 : Saturate  UpperLimit=255  LowerLimit=0
  Saturation2 : Saturate  UpperLimit=1500  LowerLimit=-1500
  Sum : Sum  Inputs=|+-
  Sum1 : Sum  Inputs=-+|
  Sum2 : Sum  Inputs=++|
  Sum4 : Sum  Inputs=++|
  phi : Constant  Value=128
  pitching controller : simulink/Continuous/PID Controller  Controller=PID  TimeDomain=Continuous-time  SampleTime=1  IntegratorMethod=Forward Euler  FilterMethod=Forward Euler  Form=Parallel  P=25  I=10  D=20  N=100  InitialConditionSource=internal  InitialConditionForIntegrator=0  InitialConditionForFilter=0  ExternalReset=none  LimitOutput=on  UpperSaturationLimit=128  LowerSaturationLimit=-128  LinearizeAsGain=off  AntiWindupMode=clamping  Kb=1  TrackingMode=off  Kt=1  PParamMin=[]  PParamMax=[]  IParamMin=[]  IParamMax=[]  DParamMin=[]  DParamMax=[]  NParamMin=[]  NParamMax=[]  KbParamMin=[]  KbParamMax=[]  KtParamMin=[]  KtParamMax=[]  POutMin=[]  POutMax=[]  IOutMin=[]  IOutMax=[]  DOutMin=[]  DOutMax=[]  NOutMin=[]  NOutMax=[]  KbOutMin=[]  KbOutMax=[]  KtOutMin=[]  KtOutMax=[]  IntegratorOutMin=[]  IntegratorOutMax=[]  FilterOutMin=[]  FilterOutMax=[]  SumOutMin=[]  SumOutMax=[]  SumI1OutMin=[]  SumI1OutMax=[]  SumI2OutMin=[]  SumI2OutMax=[]  SumI3OutMin=[]  SumI3OutMax=[]  SumDOutMin=[]  SumDOutMax=[]  SaturationOutMin=[]  SaturationOutMax=[]  IntegratorContinuousStateAttributes=''  IntegratorStateMustResolveToSignalObject=off  IntegratorRTWStateStorageClass=Auto  FilterContinuousStateAttributes=''  FilterStateMustResolveToSignalObject=off  FilterRTWStateStorageClass=Auto
  rpsi : Constant  Value=128
  set_vx : Constant  Value=0
  set_vy : Constant  Value=0
  theta : Constant  Value=128
  yawing controller1 : simulink/Continuous/PID Controller  Controller=PD  TimeDomain=Continuous-time  SampleTime=1  IntegratorMethod=Forward Euler  FilterMethod=Forward Euler  Form=Parallel  P=20  I=171.290943041777  D=50  N=50  InitialConditionSource=internal  InitialConditionForIntegrator=0  InitialConditionForFilter=0  ExternalReset=none  LimitOutput=off  UpperSaturationLimit=inf  LowerSaturationLimit=-inf  LinearizeAsGain=off  AntiWindupMode=none  Kb=1  TrackingMode=off  Kt=1  PParamMin=[]  PParamMax=[]  IParamMin=[]  IParamMax=[]  DParamMin=[]  DParamMax=[]  NParamMin=[]  NParamMax=[]  KbParamMin=[]  KbParamMax=[]  KtParamMin=[]  KtParamMax=[]  POutMin=[]  POutMax=[]  IOutMin=[]  IOutMax=[]  DOutMin=[]  DOutMax=[]  NOutMin=[]  NOutMax=[]  KbOutMin=[]  KbOutMax=[]  KtOutMin=[]  KtOutMax=[]  IntegratorOutMin=[]  IntegratorOutMax=[]  FilterOutMin=[]  FilterOutMax=[]  SumOutMin=[]  SumOutMax=[]  SumI1OutMin=[]  SumI1OutMax=[]  SumI2OutMin=[]  SumI2OutMax=[]  SumI3OutMin=[]  SumI3OutMax=[]  SumDOutMin=[]  SumDOutMax=[]  SaturationOutMin=[]  SaturationOutMax=[]  IntegratorContinuousStateAttributes=''  IntegratorStateMustResolveToSignalObject=off  IntegratorRTWStateStorageClass=Auto  FilterContinuousStateAttributes=''  FilterStateMustResolveToSignalObject=off  FilterRTWStateStorageClass=Auto
  Out : Outport
  wires:
  Mux1/1 -> Out/1
  set_vx/1 -> Sum/1
  Sum4/1 -> Saturation/1
  Sum2/1 -> Saturation1/1
  phi/1 -> Sum4/1
  set_vy/1 -> Sum1/2
  theta/1 -> Sum2/1
  vy_return/1 -> Sum1/1
  vx_return/1 -> Sum/2
  " rolling controller"/1 -> Sum4/2
  rpsi/1 -> Mux1/3
  Sum1/1 -> " rolling controller"/1
  Sum/1 -> pitching controller/1
  pitching controller/1 -> Sum2/2
  Add/1 -> yawing controller1/1
  yawing controller1/1 -> Saturation2/1  "zdotdot"
  Saturation/1 -> Mux1/1
  Saturation1/1 -> Mux1/2
  Saturation2/1 -> Mux1/4
  height_return/1 -> Add/2
  set_height/1 -> Add/1

== system System_Design_Quadrocopter_2012/Subsystem/coordination system shifting ==
  "vx, vy, rpsi" : Inport
  Demux2 : Demux  Outputs=3
  Integrator1 : Integrator
  coordination system shifting : MATLAB Function  TreatAsAtomicUnit=on
  Vx : Outport
  Vy : Outport  Port=2
  wires:
  Integrator1/1 -> coordination system shifting/3(yaw)
  Demux2/3 -> Integrator1/1
  Demux2/2 -> coordination system shifting/2(yin)
  Demux2/1 -> coordination system shifting/1(xin)
  "vx, vy, rpsi"/1 -> Demux2/1
  coordination system shifting/1(x) -> Vx/1  "x"
  coordination system shifting/2(y) -> Vy/1  "y"

== system System_Design_Quadrocopter_2012/Sensors1/acc_ax_sensor/Sensor Noise ==
  Enable : EnablePort  PropagateVarSize=During execution
  Random Number3 : RandomNumber  Variance=0.0003  Seed=676  SampleTime=Ts
  Noise : Outport
  wires:
  Random Number3/1 -> Noise/1

== system System_Design_Quadrocopter_2012/Sensors1/acc_ay_sensor/Sensor Noise ==
  Enable : EnablePort  PropagateVarSize=During execution
  Random Number2 : RandomNumber  Variance=0.0003  Seed=4564  SampleTime=0.01
  Noise : Outport
  wires:
  Random Number2/1 -> Noise/1

== system System_Design_Quadrocopter_2012/Sensors1/rate_phi_sensor/Sensor Noise ==
  Enable : EnablePort  PropagateVarSize=During execution
  Random Number1 : RandomNumber  Variance=3.0462e-8  Seed=45632  SampleTime=0.01
  Noise : Outport
  wires:
  Random Number1/1 -> Noise/1

== system System_Design_Quadrocopter_2012/Sensors1/rate_psi_sensor/Sensor Noise ==
  Enable : EnablePort  PropagateVarSize=During execution
  Random Number4 : RandomNumber  Variance=3.0462e-8  Seed=1634  SampleTime=0.01
  Noise : Outport
  wires:
  Random Number4/1 -> Noise/1

== system System_Design_Quadrocopter_2012/Sensors1/rate_theta_sensor/Sensor Noise ==
  Enable : EnablePort  PropagateVarSize=During execution
  Random Number5 : RandomNumber  Variance=3.0462e-8  Seed=4731  SampleTime=0.01
  Noise : Outport
  wires:
  Random Number5/1 -> Noise/1

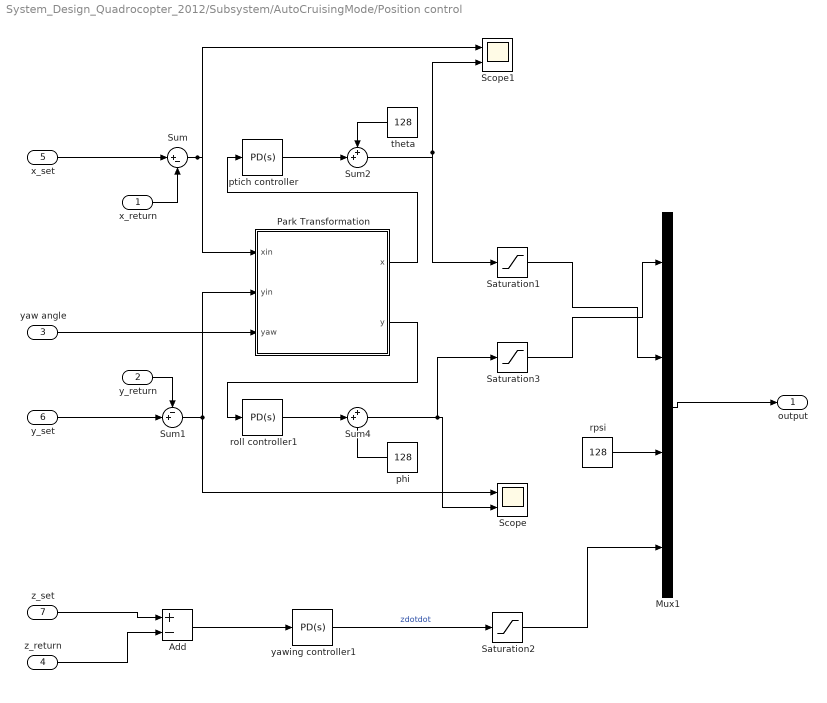
== system System_Design_Quadrocopter_2012/Subsystem/AutoCruisingMode/Position control ==
  x_return : Inport
  y_return : Inport  Port=2
  yaw angle : Inport  Port=3
  z_return : Inport  Port=4
  x_set : Inport  Port=5
  y_set : Inport  Port=6
  z_set : Inport  Port=7
  Add : Sum  Inputs=+-
  Mux1 : Mux
  Park Transformation : MATLAB Function  TreatAsAtomicUnit=on
  Saturation1 : Saturate  UpperLimit=255  LowerLimit=0
  Saturation2 : Saturate  UpperLimit=255  LowerLimit=0
  Saturation3 : Saturate  UpperLimit=255  LowerLimit=0
  Scope : Scope  NumInputPorts=2
      settings: YMin=-5~-5  YMax=5~5  SaveName=ScopeData33
  Scope1 : Scope  NumInputPorts=2
      settings: YMin=-5~-5  YMax=5~5  SaveName=ScopeData17
  Sum : Sum  Inputs=|+-
  Sum1 : Sum  Inputs=-+|
  Sum2 : Sum  Inputs=++|
  Sum4 : Sum  Inputs=++|
  phi : Constant  Value=128
  ptich controller : simulink/Continuous/PID Controller  Controller=PD  TimeDomain=Continuous-time  SampleTime=1  IntegratorMethod=Forward Euler  FilterMethod=Forward Euler  Form=Parallel  P=10  I=10  D=50  N=50  InitialConditionSource=internal  InitialConditionForIntegrator=0  InitialConditionForFilter=0  ExternalReset=none  LimitOutput=on  UpperSaturationLimit=128  LowerSaturationLimit=-128  LinearizeAsGain=off  AntiWindupMode=clamping  Kb=1  TrackingMode=off  Kt=1  PParamMin=[]  PParamMax=[]  IParamMin=[]  IParamMax=[]  DParamMin=[]  DParamMax=[]  NParamMin=[]  NParamMax=[]  KbParamMin=[]  KbParamMax=[]  KtParamMin=[]  KtParamMax=[]  POutMin=[]  POutMax=[]  IOutMin=[]  IOutMax=[]  DOutMin=[]  DOutMax=[]  NOutMin=[]  NOutMax=[]  KbOutMin=[]  KbOutMax=[]  KtOutMin=[]  KtOutMax=[]  IntegratorOutMin=[]  IntegratorOutMax=[]  FilterOutMin=[]  FilterOutMax=[]  SumOutMin=[]  SumOutMax=[]  SumI1OutMin=[]  SumI1OutMax=[]  SumI2OutMin=[]  SumI2OutMax=[]  SumI3OutMin=[]  SumI3OutMax=[]  SumDOutMin=[]  SumDOutMax=[]  SaturationOutMin=[]  SaturationOutMax=[]  IntegratorContinuousStateAttributes=''  IntegratorStateMustResolveToSignalObject=off  IntegratorRTWStateStorageClass=Auto  FilterContinuousStateAttributes=''  FilterStateMustResolveToSignalObject=off  FilterRTWStateStorageClass=Auto
  roll controller1 : simulink/Continuous/PID Controller  Controller=PD  TimeDomain=Continuous-time  SampleTime=1  IntegratorMethod=Forward Euler  FilterMethod=Forward Euler  Form=Parallel  P=10  I=10  D=50  N=50  InitialConditionSource=internal  InitialConditionForIntegrator=0  InitialConditionForFilter=0  ExternalReset=none  LimitOutput=on  UpperSaturationLimit=128  LowerSaturationLimit=-128  LinearizeAsGain=off  AntiWindupMode=clamping  Kb=1  TrackingMode=off  Kt=1  PParamMin=[]  PParamMax=[]  IParamMin=[]  IParamMax=[]  DParamMin=[]  DParamMax=[]  NParamMin=[]  NParamMax=[]  KbParamMin=[]  KbParamMax=[]  KtParamMin=[]  KtParamMax=[]  POutMin=[]  POutMax=[]  IOutMin=[]  IOutMax=[]  DOutMin=[]  DOutMax=[]  NOutMin=[]  NOutMax=[]  KbOutMin=[]  KbOutMax=[]  KtOutMin=[]  KtOutMax=[]  IntegratorOutMin=[]  IntegratorOutMax=[]  FilterOutMin=[]  FilterOutMax=[]  SumOutMin=[]  SumOutMax=[]  SumI1OutMin=[]  SumI1OutMax=[]  SumI2OutMin=[]  SumI2OutMax=[]  SumI3OutMin=[]  SumI3OutMax=[]  SumDOutMin=[]  SumDOutMax=[]  SaturationOutMin=[]  SaturationOutMax=[]  IntegratorContinuousStateAttributes=''  IntegratorStateMustResolveToSignalObject=off  IntegratorRTWStateStorageClass=Auto  FilterContinuousStateAttributes=''  FilterStateMustResolveToSignalObject=off  FilterRTWStateStorageClass=Auto
  rpsi : Constant  Value=128
  theta : Constant  Value=128
  yawing controller1 : simulink/Continuous/PID Controller  Controller=PD  TimeDomain=Continuous-time  SampleTime=1  IntegratorMethod=Forward Euler  FilterMethod=Forward Euler  Form=Parallel  P=20  I=171.290943041777  D=50  N=50  InitialConditionSource=internal  InitialConditionForIntegrator=0  InitialConditionForFilter=0  ExternalReset=none  LimitOutput=off  UpperSaturationLimit=inf  LowerSaturationLimit=-inf  LinearizeAsGain=off  AntiWindupMode=none  Kb=1  TrackingMode=off  Kt=1  PParamMin=[]  PParamMax=[]  IParamMin=[]  IParamMax=[]  DParamMin=[]  DParamMax=[]  NParamMin=[]  NParamMax=[]  KbParamMin=[]  KbParamMax=[]  KtParamMin=[]  KtParamMax=[]  POutMin=[]  POutMax=[]  IOutMin=[]  IOutMax=[]  DOutMin=[]  DOutMax=[]  NOutMin=[]  NOutMax=[]  KbOutMin=[]  KbOutMax=[]  KtOutMin=[]  KtOutMax=[]  IntegratorOutMin=[]  IntegratorOutMax=[]  FilterOutMin=[]  FilterOutMax=[]  SumOutMin=[]  SumOutMax=[]  SumI1OutMin=[]  SumI1OutMax=[]  SumI2OutMin=[]  SumI2OutMax=[]  SumI3OutMin=[]  SumI3OutMax=[]  SumDOutMin=[]  SumDOutMax=[]  SaturationOutMin=[]  SaturationOutMax=[]  IntegratorContinuousStateAttributes=''  IntegratorStateMustResolveToSignalObject=off  IntegratorRTWStateStorageClass=Auto  FilterContinuousStateAttributes=''  FilterStateMustResolveToSignalObject=off  FilterRTWStateStorageClass=Auto
  output : Outport
  wires:
  y_set/1 -> Sum1/2
  x_set/1 -> Sum/1
  ptich controller/1 -> Sum2/2
  Sum/1 -> Park Transformation/1(xin), Scope1/1
  Sum1/1 -> Scope/1, Park Transformation/2(yin)
  roll controller1/1 -> Sum4/2
  x_return/1 -> Sum/2
  y_return/1 -> Sum1/1
  theta/1 -> Sum2/1
  phi/1 -> Sum4/1
  Sum2/1 -> Scope1/2, Saturation1/1
  Sum4/1 -> Scope/2, Saturation3/1
  yaw angle/1 -> Park Transformation/3(yaw)
  Park Transformation/2(y) -> roll controller1/1
  Park Transformation/1(x) -> ptich controller/1
  z_return/1 -> Add/2
  Add/1 -> yawing controller1/1
  yawing controller1/1 -> Saturation2/1  "zdotdot"
  z_set/1 -> Add/1
  Mux1/1 -> output/1
  rpsi/1 -> Mux1/3
  Saturation2/1 -> Mux1/4
  Saturation1/1 -> Mux1/2
  Saturation3/1 -> Mux1/1

== matlab function Subsystem/Cutoff switch/cutoff switch ==
  data: y output double
function y = fcn()
%#codegen
coder.extrinsic('get_param');
if strcmp(get_param('System_Design_Quadrocopter_2012/Switch1','sw'), '1')
    y=0;
  
else
    y=1;
  %set_param([gcb '/Manual Switch'], 'sw', '0');
  %set_param(gcb, 'MaskDisplay', 'fprintf(''False'')');
end

== matlab function Subsystem/coordination system shifting/coordination system shifting ==
  data: x output double; y output double; xin input double; yin input double; yaw input double
function [x,y] = fcn(xin, yin, yaw)
%#codegen
x =cos(yaw)*xin + sin(yaw)*yin;
y = -sin(yaw)*xin + cos(yaw)*yin;

== matlab function Subsystem/hovering height setting ==
  data: Switch1 input double; height input double; h output double
function h = fcn(Switch1,height)
h=0;
persistent b;
persistent flag;
if isempty(b)
    b=0;
end

if isempty(flag)
    flag=0;
end
if Switch1==1&&flag==0;
    flag=1;
    b=height;
else if Switch1==0
    flag=0;
    b=0;
    end
end
h=b;

== matlab function Subsystem/AutoCruisingMode/Position control/Park Transformation ==
  data: x output double; y output double; xin input double; yin input double; yaw input double
function [x,y] = fcn(xin, yin, yaw)
%#codegen
x =cos(yaw)*xin + sin(yaw)*yin;
y = -sin(yaw)*xin + cos(yaw)*yin;
